simulink model "sensors"  (R2018b)
settings: Solver=VariableStepAuto  StartTime=0.0  StopTime=480  FixedStep=1e-3  RelTol=1e-3
libraries: simulink x2
settings Model: Creator=César  LastModifiedBy=César

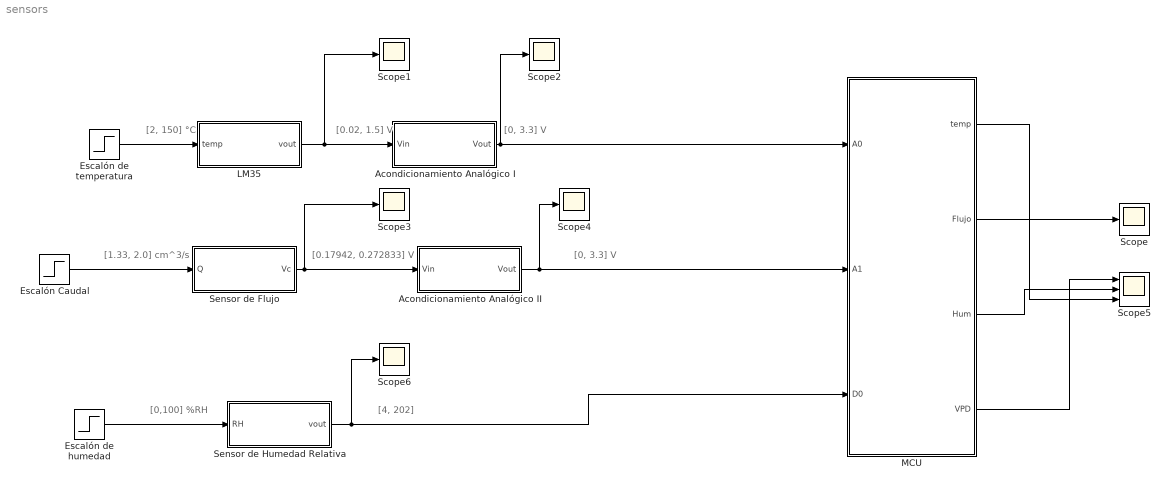
== system sensors ==
  note: [0, 3.3] V
  note: [0.02, 1.5] V
  note: [2, 150] °C
  note: [1.33, 2.0] cm^3/s
  note: [0.17942, 0.272833] V
  note: [0, 3.3] V
  note: [0,100] %RH
  note: [4, 202]
  Acondicionamiento Analógico I : Subsystem  Tag=LM35  Description=Temperature Sensor
  Acondicionamiento Analógico II : Subsystem  Tag=LM35  Description=Temperature Sensor
  Escalón Caudal : Step  After=2.0  SampleTime=0
  "Escalón de humedad " : Step  After=70  SampleTime=0
  Escalón de temperatura : Step  Before=2  After=25  SampleTime=0
  LM35 : Subsystem  Tag=LM35  Description=Temperature Sensor
  MCU : Subsystem  Tag=LM35  Description=Temperature Sensor
  Scope{,1..4,6} (6 alike) : Scope
  Scope5 : Scope  NumInputPorts=3
  Sensor de Flujo : Subsystem  Tag=LM35  Description=Temperature Sensor
  Sensor de Humedad Relativa : Subsystem  Tag=LM35  Description=Temperature Sensor
  wires:
  Escalón de temperatura/1 -> LM35/1("temp ")
  MCU/1("temp ") -> Scope5/3
  Acondicionamiento Analógico I/1("Vout ") -> MCU/1("A0 "), Scope2/1
  Sensor de Humedad Relativa/1("vout ") -> Scope6/1, MCU/3("D0 ")
  "Escalón de humedad "/1 -> Sensor de Humedad Relativa/1("RH ")
  Escalón Caudal/1 -> Sensor de Flujo/1("Q ")
  Acondicionamiento Analógico II/1("Vout ") -> MCU/2("A1 "), Scope4/1
  Sensor de Flujo/1("Vc ") -> Acondicionamiento Analógico II/1("Vin "), Scope3/1
  MCU/4(VPD) -> Scope5/1
  MCU/3("Hum ") -> Scope5/2
  MCU/2(Flujo) -> Scope/1
  LM35/1("vout ") -> Acondicionamiento Analógico I/1("Vin "), Scope1/1

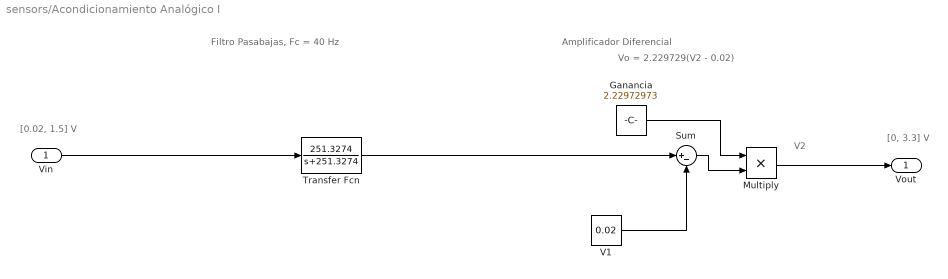
== system sensors/Acondicionamiento Analógico I ==
  note: Vo = 2.229729(V2 - 0.02)
  note: V2
  note: [0, 3.3] V
  note: Amplificador Diferencial
  note: [0.02, 1.5] V
  note: Filtro Pasabajas, Fc = 40 Hz
  "Vin " : Inport
  "Ganancia " : Constant  Value=2.22972973
  Multiply : Product
  Sum : Sum  Inputs=|+-
  Transfer Fcn : TransferFcn  Numerator=[251.3274]  Denominator=[1 251.3274]
  V1 : Constant  Value=0.02
  "Vout " : Outport
  wires:
  V1/1 -> Sum/2
  "Ganancia "/1 -> Multiply/1
  Sum/1 -> Multiply/2
  Multiply/1 -> "Vout "/1
  "Vin "/1 -> Transfer Fcn/1
  Transfer Fcn/1 -> Sum/1

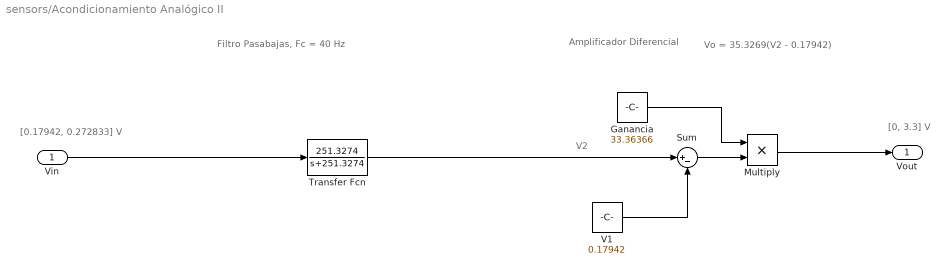
== system sensors/Acondicionamiento Analógico II ==
  note: Vo = 35.3269(V2 - 0.17942)
  note: V2
  note: [0, 3.3] V
  note: Amplificador Diferencial
  note: [0.17942, 0.272833] V
  note: Filtro Pasabajas, Fc = 40 Hz
  "Vin " : Inport
  "Ganancia " : Constant  Value=33.36366
  Multiply : Product
  Sum : Sum  Inputs=|+-
  Transfer Fcn : TransferFcn  Numerator=[251.3274]  Denominator=[1 251.3274]
  V1 : Constant  Value=0.17942
  "Vout " : Outport
  wires:
  Multiply/1 -> "Vout "/1
  V1/1 -> Sum/2
  "Ganancia "/1 -> Multiply/1
  Sum/1 -> Multiply/2
  "Vin "/1 -> Transfer Fcn/1
  Transfer Fcn/1 -> Sum/1

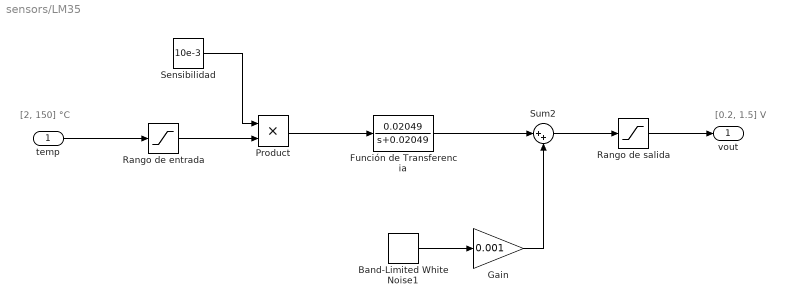
== system sensors/LM35 ==
  note: [0.2, 1.5] V
  note: [2, 150] °C
  "temp " : Inport
  Band-Limited White Noise1 : simulink/Sources/Band-Limited White Noise  Cov=[0.01]  Ts=1/60  seed=[23341]
  Función de Transferencia : TransferFcn  Numerator=[0.02049]  Denominator=[1 0.02049]
  Gain : Gain  Gain=0.001
  Product : Product
  Rango de entrada : Saturate  UpperLimit=150  LowerLimit=2
  Rango de salida : Saturate  UpperLimit=1.5  LowerLimit=0.2
  Sensibilidad : Constant  Value=10e-3
  Sum2 : Sum  Inputs=|++
  "vout " : Outport
  wires:
  Sensibilidad/1 -> Product/1
  Product/1 -> Función de Transferencia/1
  Band-Limited White Noise1/1 -> Gain/1
  Función de Transferencia/1 -> Sum2/1
  "temp "/1 -> Rango de entrada/1
  Rango de entrada/1 -> Product/2
  Sum2/1 -> Rango de salida/1
  Rango de salida/1 -> "vout "/1
  Gain/1 -> Sum2/2

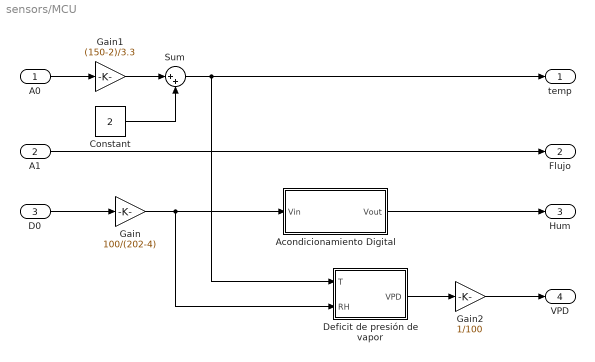
== system sensors/MCU ==
  "A0 " : Inport
  "A1 " : Inport  Port=2
  "D0 " : Inport  Port=3
  "Acondicionamiento Digital " : Subsystem  Tag=LM35  Description=Temperature Sensor
  Constant : Constant  Value=2
  Deficit de presión de vapor : MATLAB Function  TreatAsAtomicUnit=on
  Gain : Gain  Gain=100/(202-4)
  Gain1 : Gain  Gain=(150-2)/3.3
  Gain2 : Gain  Gain=1/100
  Sum : Sum  Inputs=|++
  "temp " : Outport
  Flujo : Outport  Port=2
  "Hum " : Outport  Port=3
  VPD : Outport  Port=4
  wires:
  Sum/1 -> "temp "/1, Deficit de presión de vapor/1(T)
  "Acondicionamiento Digital "/1("Vout ") -> "Hum "/1
  "A1 "/1 -> Flujo/1
  "D0 "/1 -> Gain/1
  Gain/1 -> Deficit de presión de vapor/2(RH), "Acondicionamiento Digital "/1("Vin ")
  "A0 "/1 -> Gain1/1
  Deficit de presión de vapor/1(VPD) -> Gain2/1
  Gain2/1 -> VPD/1
  Gain1/1 -> Sum/1
  Constant/1 -> Sum/2

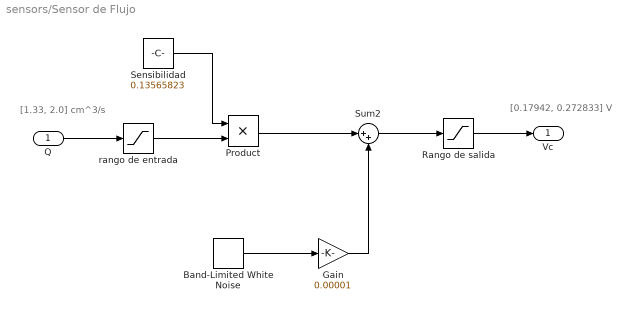
== system sensors/Sensor de Flujo ==
  note: [1.33, 2.0] cm^3/s
  note: [0.17942, 0.272833] V
  "Q " : Inport
  Band-Limited White Noise : simulink/Sources/Band-Limited White Noise  Cov=[0.01]  Ts=0.1  seed=[23341]
  Gain : Gain  Gain=0.00001
  Product : Product
  Rango de salida : Saturate  UpperLimit=0.28  LowerLimit=0.16
  Sensibilidad : Constant  Value=0.13565823
  Sum2 : Sum  Inputs=|++
  rango de entrada : Saturate  UpperLimit=2.0  LowerLimit=1.32
  "Vc " : Outport
  wires:
  Sensibilidad/1 -> Product/1
  "Q "/1 -> rango de entrada/1
  rango de entrada/1 -> Product/2
  Sum2/1 -> Rango de salida/1
  Product/1 -> Sum2/1
  Gain/1 -> Sum2/2
  Band-Limited White Noise/1 -> Gain/1
  Rango de salida/1 -> "Vc "/1

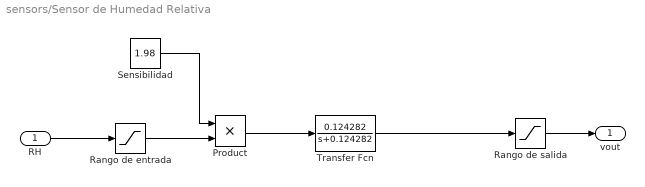
== system sensors/Sensor de Humedad Relativa ==
  "RH " : Inport
  Product : Product
  Rango de entrada : Saturate  UpperLimit=100  LowerLimit=0
  Rango de salida : Saturate  UpperLimit=255  LowerLimit=0
  Sensibilidad : Constant  Value=1.98
  Transfer Fcn : TransferFcn  Numerator=[0.124282]  Denominator=[1 0.124282]
  "vout " : Outport
  wires:
  Product/1 -> Transfer Fcn/1
  Sensibilidad/1 -> Product/1
  "RH "/1 -> Rango de entrada/1
  Rango de entrada/1 -> Product/2
  Rango de salida/1 -> "vout "/1
  Transfer Fcn/1 -> Rango de salida/1

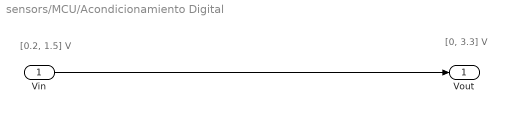
== system sensors/MCU/Acondicionamiento Digital  ==
  note: [0, 3.3] V
  note: [0.2, 1.5] V
  "Vin " : Inport
  "Vout " : Outport
  wires:
  "Vin "/1 -> "Vout "/1

== matlab function sensors/MCU/Deficit de presión de vapor ==
  data: T input; VPD output; RH input
function VPD = fcn(T,RH)

VPD = exp(6.41+(0.0727*T)-(3e-4*(T^2))+(1.18e-6*(T^3))-(3.86e-9*(T^4)))*(1-(RH/100));
